simulink model "Boost"  (Simulink 6.1)
settings: Solver=ode23tb  StartTime=0.0  StopTime=3e-2  RelTol=1e-3  AbsTol=1e-3
libraries: powerlib x7
settings Model: Creator=dkennedy  LastModifiedBy=ThinkPad  ExtModeTrigMode=oneshot  ExtModeArmWhenConnect=off  ExtModeAutoUpdateStatusClock=off
settings DataIOCC: LimitDataPoints=off  SignalLoggingName=sigsOut
settings OptimizationCC: BlockReduction=off  BooleanDataType=off
settings HardwareCC: TargetUnknown=on

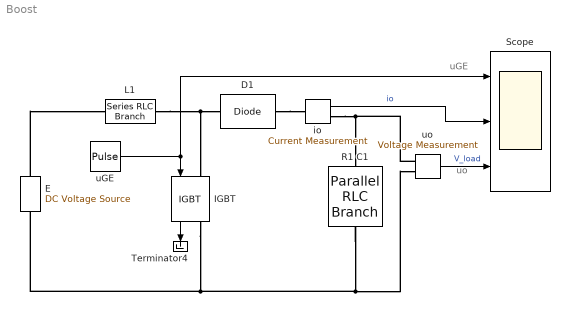
== system Boost ==
  note: uo
  note: uGE
  D1 : powerlib/Power Electronics/Diode  Ron=0.05  Lon=0.1e-6  Vf=0.8  IC=10  Rs=inf  Cs=inf  Measurements=off
  E : powerlib/Electrical Sources/DC Voltage Source  Description=source block  Orientation=up  Amplitude=100  Measurements=None
      settings: AttributesFormatString=\n
  IGBT : powerlib/Power Electronics/IGBT  Orientation=down  Ron=0.01  Lon=1e-6  Vf=1  Tf=1e-6  Tt=1e-6  IC=0  Rs=1000  Cs=1e-7  Measurements=on
      settings: AttributesFormatString=\n
  L1 : powerlib/Elements/Series RLC Branch  PhysicalDomain=powersysdomain  SubClassName=unknown  LeftPortType=p1  RightPortType=p1  LConnTagsString=__new0  RConnTagsString=__new0  Resistance=0  Inductance=20e-3  Capacitance=inf  Measurements=None
  R1 C1 : powerlib/Elements/Parallel RLC Branch  Orientation=down  PhysicalDomain=powersysdomain  SubClassName=unknown  LeftPortType=p1  RightPortType=p1  LConnTagsString=a  RConnTagsString=__new0  Resistance=25  Inductance=inf  Capacitance=100e-06  Measurements=None
  Scope : Scope  NumInputPorts=3
      settings: TimeRange=0.01  YMin=-1~-10~0  YMax=2~100~500  SaveName=var  MaxDataPoints=50000
  Terminator4 : Terminator
      settings: Orientation=down
  io : powerlib/Measurements/Current Measurement  PhasorSimulation=off  OutputType=Complex  PSBequivalent=0
  uGE : DiscretePulseGenerator  PulseType=Time based  Period=1e-3  PulseWidth=70
  uo : powerlib/Measurements/Voltage Measurement  Tag=PoWeRsYsTeMmEaSuReMeNt  PhasorSimulation=off  OutputType=Magnitude  PSBequivalent=0
  wires:
  io/1 -> Scope/2  "io"
  uGE/1 -> IGBT/1, Scope/1
  uo/1 -> Scope/3  "V_load"
  IGBT/1 -> Terminator4/1
  connections:
  uo/LConn1 -- R1 C1/LConn1 -- io/RConn1
  R1 C1/RConn1 -- uo/LConn2 -- E/LConn1 -- IGBT/RConn1
  E/RConn1 -- L1/LConn1
  L1/RConn1 -- D1/LConn1 -- IGBT/LConn1
  D1/RConn1 -- io/LConn1
